simulink model "speed_obs_pll_Harness1"  (R2023a)
settings: configuration reference "config" (kept outside this file)
model workspace (MAT data in the model file):
  enc_line_inv_p_n = Simulink.Parameter
  enc_line_inv_p_n.Value = 0.00025
  enc_line_inv_p_n.Description = '编码器分辨率 倒数'
  enc_line_inv_p_n.DataType = 'single'
  enc_line_inv_p_n.Complexity = 'real'
  enc_line_inv_p_n.Dimensions = [1 1]
  tp = Simulink.Parameter
  tp.Value = 0.0001
  tp.Description = '位置环速度环执行周期'
  tp.DataType = 'single'
  tp.Complexity = 'real'
  tp.Dimensions = [1 1]
  wn_Hz = Simulink.Parameter
  wn_Hz.Value = 1600
  wn_Hz.Description = '滤波器截止频率  rad
    | '
  wn_Hz.DataType = 'auto'
  wn_Hz.Complexity = 'real'
  wn_Hz.Dimensions = [1 1]
libraries: simulink x2
settings Model: DataDictionary=model_config.sldd  ParameterArgumentNames=enc_line_inv_p_n,tp  Creator=Administrator  LastModifiedBy=Administrator
settings ConfigSetRef: SourceName=config

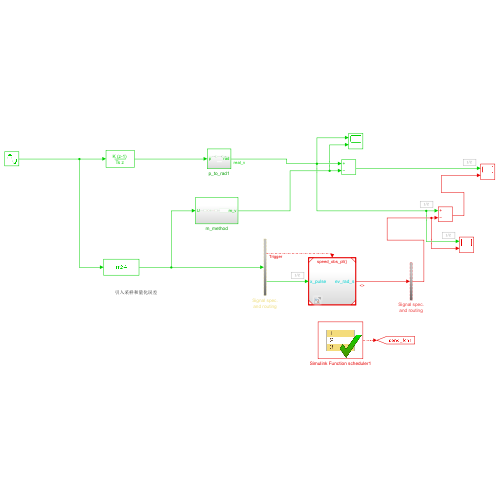
[thumbnail: Simulink's stored preview of the top-level diagram]
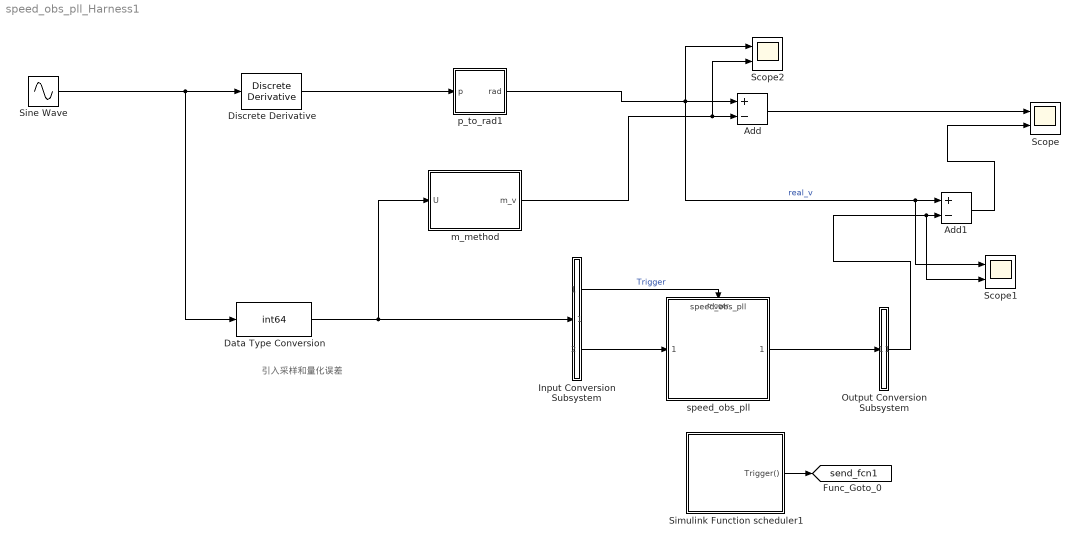
== system speed_obs_pll_Harness1 ==
  note: 引入采样和量化误差
  Add : Sum  Inputs=+-
  Add1 : Sum  Inputs=+-
  Data Type Conversion : DataTypeConversion  OutDataTypeStr=int64  SaturateOnIntegerOverflow=off  RndMeth=Floor
  Discrete Derivative : simulink/Discrete/Discrete Derivative  gainval=1.0  ICPrevScaledInput=0.0  OutMin=[]  OutMax=[]  OutDataType=fixdt(1, 16)  OutScaling=2^-10  DoSatur=off
  Input Conversion Subsystem : Subsystem  Tag=__SLT_ICS__  Description=|
      | Signal spec.
      | and routing
      settings: AttributesFormatString=%<Description>
  Output Conversion Subsystem : Subsystem  Tag=__SLT_OCS__  Description=|
      | Signal spec.
      | and routing
      settings: AttributesFormatString=%<Description>
  Scope : Scope  NumInputPorts=2
  Scope1 : Scope  NumInputPorts=2
  Scope2 : Scope  NumInputPorts=2
  Simulink Function scheduler1 : Test Sequence  Tag=__SLT_FCN_CALL__  TreatAsAtomicUnit=on
  Sine Wave : Sin  Amplitude=10000  SampleTime=10e-5
  m_method : Subsystem
  p_to_rad1 : Subsystem
  speed_obs_pll : ModelReference  ModelNameDialog=speed_obs_pll  UsingDefaultArgumentValue=0,0,0  SimulationMode=Normal  ModelReferenceVersion=2.251  TriggerPortName=Trigger  TriggerPortTriggerType=function-call  TriggerPortStatesWhenEnabling=held
  tag scope: send_fcn1=global
  wires:
  Data Type Conversion/1 -> Input Conversion Subsystem/1(Inport_1), m_method/1(U)
  Output Conversion Subsystem/1(Outport_1) -> Scope1/2, Add1/2
  Input Conversion Subsystem/2(Outport_1) -> speed_obs_pll/1
  speed_obs_pll/1 -> Output Conversion Subsystem/1(Inport_1)
  Simulink Function scheduler1/1(Trigger()) -> [send_fcn1]
  Sine Wave/1 -> Data Type Conversion/1, Discrete Derivative/1
  Discrete Derivative/1 -> p_to_rad1/1(p)
  p_to_rad1/1(rad) -> Scope2/1, Scope1/1, Add1/1, Add/1  "real_v"
  m_method/1(m_v) -> Scope2/2, Add/2
  Add/1 -> Scope/1
  Add1/1 -> Scope/2
  Input Conversion Subsystem/1(Outport_2) -> speed_obs_pll/Trigger  "Trigger"

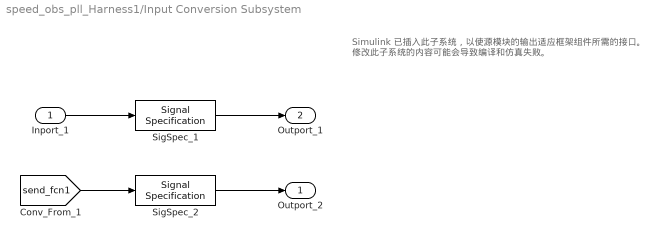
== system speed_obs_pll_Harness1/Input Conversion Subsystem ==
  note: Simulink 已插入此子系统，以使源模块的输出适应框架组件所需的接口。
      |  修改此子系统的内容可能会导致编译和仿真失败。
  Inport_1 : Inport
  SigSpec_1 : SignalSpecification  OutDataTypeStr=fixdt('int64')  Dimensions=[1]
  SigSpec_2 : SignalSpecification
  Outport_2 : Outport
  Outport_1 : Outport  Port=2
  wires:
  SigSpec_1/1 -> Outport_1/1
  Inport_1/1 -> SigSpec_1/1
  SigSpec_2/1 -> Outport_2/1
  [send_fcn1] -> SigSpec_2/1

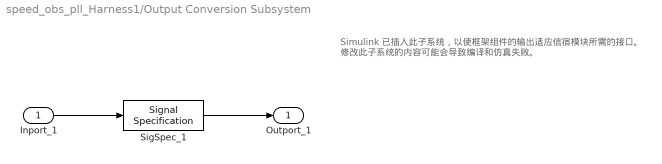
== system speed_obs_pll_Harness1/Output Conversion Subsystem ==
  note: Simulink 已插入此子系统，以使框架组件的输出适应信宿模块所需的接口。
      |  修改此子系统的内容可能会导致编译和仿真失败。
  Inport_1 : Inport
  SigSpec_1 : SignalSpecification  OutDataTypeStr=single  Dimensions=[1]
  Outport_1 : Outport
  wires:
  Inport_1/1 -> SigSpec_1/1
  SigSpec_1/1 -> Outport_1/1

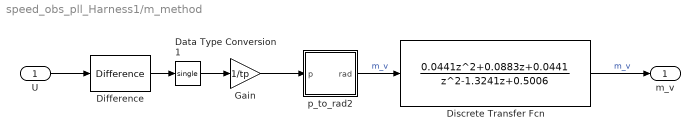
== system speed_obs_pll_Harness1/m_method ==
  U : Inport
  Data Type Conversion1 : DataTypeConversion  OutDataTypeStr=single  SaturateOnIntegerOverflow=off  RndMeth=Floor
  Difference : simulink/Discrete/Difference  ICPrevInput=0.0  OutMin=[]  OutMax=[]  OutDataType=fixdt(1, 16)  OutScaling=2^-10  DoSatur=off
  Discrete Transfer Fcn : DiscreteTransferFcn  Numerator=[0.0441 0.0883 0.0441]  Denominator=[1 -1.3241 0.5006]
  Gain : Gain  Gain=1/tp
  p_to_rad2 : Subsystem
  m_v : Outport
  wires:
  U/1 -> Difference/1
  p_to_rad2/1(rad) -> Discrete Transfer Fcn/1  "m_v"
  Difference/1 -> Data Type Conversion1/1
  Gain/1 -> p_to_rad2/1(p)
  Data Type Conversion1/1 -> Gain/1
  Discrete Transfer Fcn/1 -> m_v/1  "m_v"

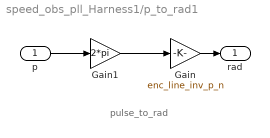
== system speed_obs_pll_Harness1/p_to_rad1 ==
  note: pulse_to_rad
  p : Inport
  Gain : Gain  Gain=enc_line_inv_p_n
  Gain1 : Gain  Gain=2*pi
  rad : Outport
  wires:
  Gain/1 -> rad/1
  Gain1/1 -> Gain/1
  p/1 -> Gain1/1

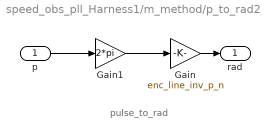
== system speed_obs_pll_Harness1/m_method/p_to_rad2 ==
  note: pulse_to_rad
  p : Inport
  Gain : Gain  Gain=enc_line_inv_p_n
  Gain1 : Gain  Gain=2*pi
  rad : Outport
  wires:
  p/1 -> Gain1/1
  Gain1/1 -> Gain/1
  Gain/1 -> rad/1

== stateflow chart speed_obs_pll_Harness1/Simulink Function scheduler1 ==
  settings: updateMethod=DISCRETE  sampleTime=1.0E-5
  state Run
    num = 0;
    send(Trigger);
  state step_1
    num = num +1;
  state step_2
    num = 0;
    send(Trigger);
  (default) -> Run
  Run -> step_1 : [
      | true
      | ]
  step_1 -> step_2 : [
      | num >8
      | ]
  step_2 -> step_1 : [
      | true
      | ]
  data: num local
  events: Trigger output FUNCTION_CALL_EVENT
